simulink model "problem9_bldc"  (R2020b)
settings: Solver=VariableStepAuto  StartTime=0.0  StopTime=10.0  RelTol=1e-3
PostLoadFcn:
  | J=0.01;
  | R=1;
  | L=0.5;
  | b=0.1;
  | Ke=0.01;
  | Kt=0.01;
settings Model: Creator=Gopinath Murugan  LastModifiedBy=Gopinath Murugan

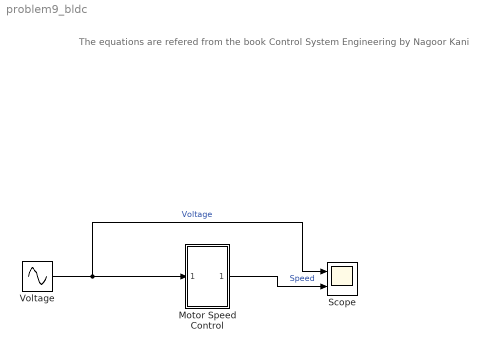
== system problem9_bldc ==
  note: The equations are refered from the book Control System Engineering by Nagoor Kani
  Motor Speed Control : Subsystem
  Scope : Scope  NumInputPorts=2
  Voltage : Sin  Amplitude=5  SampleTime=0
  wires:
  Voltage/1 -> Scope/1, Motor Speed Control/1(In1)  "Voltage"
  Motor Speed Control/1(Out1) -> Scope/2  "Speed"

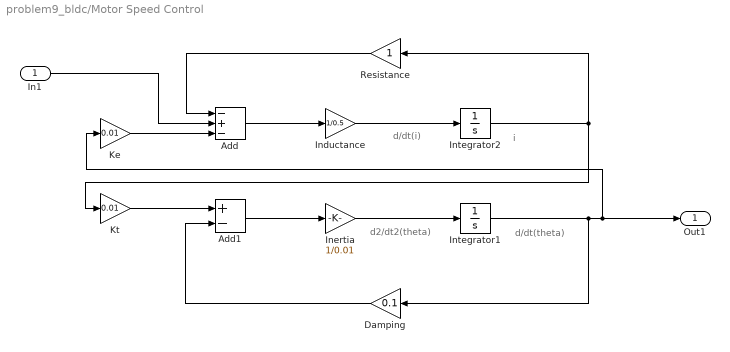
== system problem9_bldc/Motor Speed Control ==
  note: i
  note: d/dt(i)
  note: d2/dt2(theta)
  note: d/dt(theta)
  In1 : Inport
  Add : Sum  Inputs=-+-
  Add1 : Sum  Inputs=+-
  Damping : Gain  Gain=0.1
  Inductance : Gain  Gain=1/0.5
  Inertia : Gain  Gain=1/0.01
  Integrator1 : Integrator
  Integrator2 : Integrator
  Ke : Gain  Gain=0.01
  Kt : Gain  Gain=0.01
  Resistance : Gain
  Out1 : Outport
  wires:
  Inductance/1 -> Integrator2/1
  Resistance/1 -> Add/1
  Integrator2/1 -> Resistance/1, Kt/1
  Integrator1/1 -> Damping/1, Out1/1, Ke/1
  Damping/1 -> Add1/2
  Add/1 -> Inductance/1
  Ke/1 -> Add/3
  Add1/1 -> Inertia/1
  Inertia/1 -> Integrator1/1
  Kt/1 -> Add1/1
  In1/1 -> Add/2
